simulink model "nms_3Dmodel_mld"  (R2019a)
settings: Solver=ode15s  StartTime=0.0  StopTime=7  FixedStep=1e-3  RelTol=1e-3  AbsTol=1e-4  EnableMultiTasking=on
InitFcn:
  | runScripts;
undefined symbols (not defined in the file or in its folder): ankle_height, c, c_jointstop, CtrlPar_FP, CtrlPar_FP_R, CtrlPar_LL, CtrlPar_St, CtrlPar_St_R, CtrlPar_Sw, CtrlPar_Sw_R, CtrlPar_theta0, CtrlPar_Tr, CtrlPar_Tr_R, D12_F, D12_S, D12_T, D12z_T, D13_F, D1G_F, D1G_HAT, D1G_S, D1G_T, D1Gy_F, d_fBall, d_fHeel, DeltaThRef, dt, eref, FmaxBFSH, FmaxGAS, FmaxGLU, FmaxHAB, FmaxHAD, FmaxHAM, FmaxHFL, FmaxRF, FmaxSOL, FmaxTA, FmaxVAS, In_F, In_HAT, In_S, In_T, init_a_tgt, init_a_tgtR, Inx_F, Inx_HAT, Inx_S, Inx_T, Iny_F, Iny_HAT, Iny_S, Iny_T, K, k_gn, k_gt, k_pressure, leg_l, LongDelay, LongLoopDelay ... (+139)
libraries: mblibv1 x89, simulink x44, simulink_extras x38
(part 7 of 13)

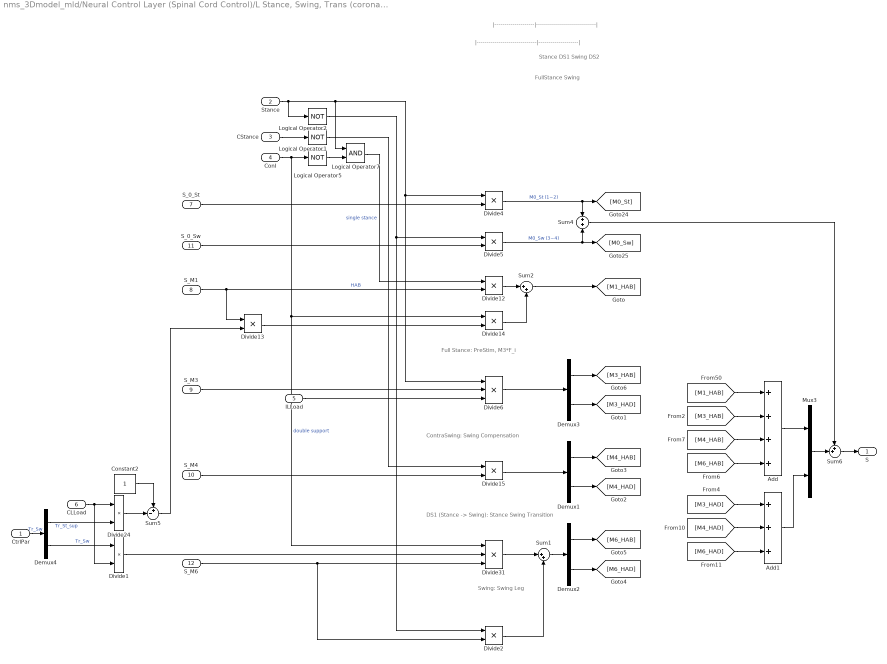
== system nms_3Dmodel_mld/Neural Control Layer (Spinal Cord Control)/L Stance, Swing, Trans (coronal) ==
  note: DS1 (Stance -> Swing):
      | Stance Swing Transition
  note: Swing:
      | Swing Leg
  note: Full Stance:
      | PreStim, M3*F_i
  note: Stance DS1 Swing DS2
  note: FullStance Swing
  note: |------------------------------|--------------------|
  note: |--------------------|------------------------------|
  note: ContraSwing:
      | Swing Compensation
  CtrlPar : Inport
  Stance : Inport  Port=2
  CStance : Inport  Port=3
  ConI : Inport  Port=4
  ILLoad : Inport  Port=5
  CLLoad : Inport  Port=6
  S_0_St : Inport  Port=7
  S_M1 : Inport  Port=8
  S_M3 : Inport  Port=9
  S_M4 : Inport  Port=10
  S_0_Sw : Inport  Port=11
  S_M6 : Inport  Port=12
  Add : Sum  Inputs=4
  Add1 : Sum  Inputs=3
  Constant2 : Constant
  Demux{1..4} (4 alike) : Demux  Outputs=2
  Divide{1..2,4..5,12..15,24} (9 alike) : Product
  Divide31 : Product  Inputs=3
  Divide6 : Product  Inputs=3
  Logical Operator1 : Logic  Operator=NOT  AllPortsSameDT=off  OutDataTypeStr=boolean
  Logical Operator2 : Logic  Operator=NOT  AllPortsSameDT=off  OutDataTypeStr=boolean
  Logical Operator5 : Logic  Operator=NOT  AllPortsSameDT=off  OutDataTypeStr=boolean
  Logical Operator7 : Logic  AllPortsSameDT=off  OutDataTypeStr=boolean
  Mux3 : Mux  Inputs=2
  Sum1 : Sum  Inputs=|++  SaturateOnIntegerOverflow=on  InputSameDT=on  OutDataTypeStr=Inherit: Same as first input
  Sum2 : Sum  Inputs=|++  SaturateOnIntegerOverflow=on  InputSameDT=on  OutDataTypeStr=Inherit: Same as first input
  Sum4 : Sum  SaturateOnIntegerOverflow=on  InputSameDT=on  OutDataTypeStr=Inherit: Same as first input
  Sum5 : Sum  Inputs=+-|  SaturateOnIntegerOverflow=on  InputSameDT=on  OutDataTypeStr=Inherit: Same as first input
  Sum6 : Sum  Inputs=++|  SaturateOnIntegerOverflow=on  InputSameDT=on  OutDataTypeStr=Inherit: Same as first input
  S : Outport  OutputWhenDisabled=reset  InitialOutput=0
  wires:
  CStance/1 -> Logical Operator1/1
  S_M4/1 -> Divide15/2
  Logical Operator1/1 -> Divide15/1
  CLLoad/1 -> Divide1/2, Divide24/1
  Divide1/1 -> Divide31/2
  ConI/1 -> Logical Operator5/1, Divide31/1, Divide14/1  "double support"
  Stance/1 -> Logical Operator2/1, Divide6/1, Divide4/1, Logical Operator7/1
  Logical Operator2/1 -> Divide2/1, Divide5/1
  Add/1 -> Mux3/1
  Add1/1 -> Mux3/2
  S_M3/1 -> Divide6/2
  ILLoad/1 -> Divide6/3
  S_0_St/1 -> Divide4/2
  S_0_Sw/1 -> Divide5/2
  Mux3/1 -> Sum6/2
  Sum6/1 -> S/1
  S_M6/1 -> Divide31/3, Divide2/2
  Divide4/1 -> Sum4/1, [M0_St]  "M0_St (1~2)"
  Divide5/1 -> Sum4/2, [M0_Sw]  "M0_Sw (3~4)"
  Divide31/1 -> Sum1/1
  Divide2/1 -> Sum1/2
  S_M1/1 -> Divide12/2, Divide13/1  "HAB"
  Divide12/1 -> Sum2/1
  Divide13/1 -> Divide14/2
  Divide14/1 -> Sum2/2
  Logical Operator5/1 -> Logical Operator7/2
  Logical Operator7/1 -> Divide12/1  "single stance"
  Divide24/1 -> Sum5/2
  Constant2/1 -> Sum5/1
  Sum5/1 -> Divide13/2
  CtrlPar/1 -> Demux4/1  "Tr_Sw"
  Demux4/1 -> Divide24/2  "Tr_St_sup"
  Demux4/2 -> Divide1/1  "Tr_Sw"
  Sum2/1 -> [M1_HAB]
  Divide6/1 -> Demux3/1
  Demux3/1 -> [M3_HAB]
  Demux3/2 -> [M3_HAD]
  Divide15/1 -> Demux1/1
  Demux1/1 -> [M4_HAB]
  Demux1/2 -> [M4_HAD]
  Demux2/1 -> [M6_HAB]
  Demux2/2 -> [M6_HAD]
  Sum1/1 -> Demux2/1
  Sum4/1 -> Sum6/1
  [M1_HAB] -> Add/1
  [M3_HAB] -> Add/2
  [M3_HAD] -> Add1/1
  [M4_HAB] -> Add/3
  [M6_HAB] -> Add/4
  [M4_HAD] -> Add1/2
  [M6_HAD] -> Add1/3

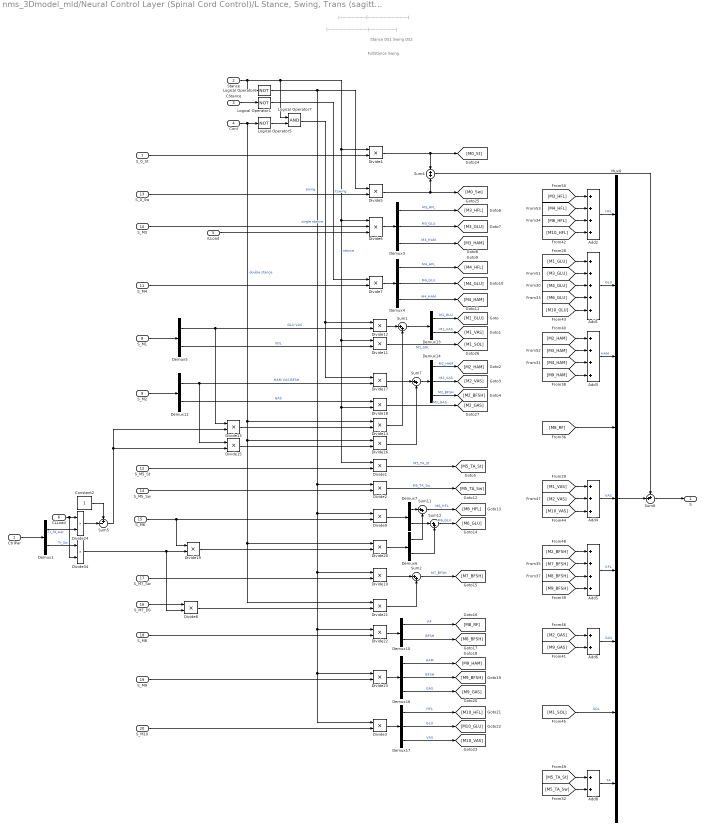
== system nms_3Dmodel_mld/Neural Control Layer (Spinal Cord Control)/L Stance, Swing, Trans (sagittal) ==
  note: Stance DS1 Swing DS2
  note: FullStance Swing
  note: |------------------------------|--------------------|
  note: |--------------------|------------------------------|
  CtrlPar : Inport
  Stance : Inport  Port=2
  CStance : Inport  Port=3
  ConI : Inport  Port=4
  ILLoad : Inport  Port=5
  CLLoad : Inport  Port=6
  S_0_St : Inport  Port=7
  S_M1 : Inport  Port=8
  S_M2 : Inport  Port=9
  S_M3 : Inport  Port=10
  S_M4 : Inport  Port=11
  S_M5_St : Inport  Port=12
  S_0_Sw : Inport  Port=13
  S_M5_Sw : Inport  Port=14
  S_M6 : Inport  Port=15
  S_M7_DS : Inport  Port=16
  S_M7_Sw : Inport  Port=17
  S_M8 : Inport  Port=18
  S_M9 : Inport  Port=19
  S_M10 : Inport  Port=20
  Add1 : Sum  Inputs=5
  Add2 : Sum  Inputs=4
  Add3 : Sum  Inputs=4
  Add4 : Sum  Inputs=3
  Add5 : Sum  Inputs=4
  Add6 : Sum  Inputs=2
  Add8 : Sum  Inputs=2
  Constant2 : Constant
  Demux{1,6..7,10,13} (5 alike) : Demux  Outputs=2
  Demux12 : Demux  Outputs=[3 1]
  Demux{3..4,14,16..17} (5 alike) : Demux  Outputs=3
  Demux5 : Demux  Outputs=[2 1]
  Divide{1..5,7..24,34} (24 alike) : Product
  Divide6 : Product  Inputs=3
  Logical Operator1 : Logic  Operator=NOT  AllPortsSameDT=off  OutDataTypeStr=boolean
  Logical Operator5 : Logic  Operator=NOT  AllPortsSameDT=off  OutDataTypeStr=boolean
  Logical Operator6 : Logic  Operator=NOT  AllPortsSameDT=off  OutDataTypeStr=boolean
  Logical Operator7 : Logic  AllPortsSameDT=off  OutDataTypeStr=boolean
  Mux6 : Mux  Inputs=9
  Sum{1..2,7,11..12} (5 alike) : Sum  Inputs=|++  SaturateOnIntegerOverflow=on  InputSameDT=on  OutDataTypeStr=Inherit: Same as first input
  Sum4 : Sum  SaturateOnIntegerOverflow=on  InputSameDT=on  OutDataTypeStr=Inherit: Same as first input
  Sum5 : Sum  Inputs=+-|  SaturateOnIntegerOverflow=on  InputSameDT=on  OutDataTypeStr=Inherit: Same as first input
  Sum6 : Sum  Inputs=++|  SaturateOnIntegerOverflow=on  InputSameDT=on  OutDataTypeStr=Inherit: Same as first input
  S : Outport  OutputWhenDisabled=reset  InitialOutput=0
  wires:
  CtrlPar/1 -> Demux1/1
  Stance/1 -> Logical Operator6/1, Logical Operator7/1, Divide4/1, Divide11/1, Divide18/2, Divide1/1, Divide6/1  "stance"
  ConI/1 -> Logical Operator5/1, Divide14/1, Divide16/1, Divide20/1, Divide21/1  "double stance"
  Logical Operator5/1 -> Logical Operator7/2
  S_M4/1 -> Divide7/2
  CStance/1 -> Logical Operator1/1
  Logical Operator1/1 -> Divide7/1  "Cswing"
  Demux1/1 -> Divide24/2  "Tr_St_sup"
  Divide24/1 -> Sum5/2
  Constant2/1 -> Sum5/1
  CLLoad/1 -> Divide24/1, Divide34/2
  Demux4/1 -> [M4_HFL]  "M4_HFL"
  Add2/1 -> Mux6/1  "HFL"
  Add1/1 -> Mux6/2  "GLU"
  Demux4/2 -> [M4_GLU]  "M4_GLU"
  Add3/1 -> Mux6/3  "HAM"
  Demux4/3 -> [M4_HAM]  "M4_HAM"
  Add4/1 -> Mux6/5  "VAS"
  Add5/1 -> Mux6/6  "KFL"
  Add6/1 -> Mux6/7  "GAS"
  Add8/1 -> Mux6/9  "TA"
  Demux1/2 -> Divide34/1  "Tr_Sw"
  Divide7/1 -> Demux4/1
  Logical Operator7/1 -> Divide12/1, Divide17/1  "single stance"
  Divide34/1 -> Divide19/2, Divide8/2
  Logical Operator6/1 -> Divide5/1, Divide2/1, Divide9/1, Divide10/1, Divide3/1, Divide23/1, Divide22/1  "swing"
  Mux6/1 -> Sum6/2
  Sum6/1 -> S/1
  Sum4/1 -> Sum6/1
  S_0_Sw/1 -> Divide5/2
  S_0_St/1 -> Divide4/2
  Divide5/1 -> [M0_Sw], Sum4/2
  Divide4/1 -> Sum4/1, [M0_St]
  S_M1/1 -> Demux5/1
  S_M2/1 -> Demux12/1
  Demux5/1 -> Divide12/2, Divide13/1  "GLU VAS"
  Demux5/2 -> Divide11/2  "SOL"
  Divide12/1 -> Sum1/1
  Divide13/1 -> Divide14/2
  Divide14/1 -> Sum1/2
  Divide16/1 -> Sum7/2
  Divide15/1 -> Divide16/2
  Sum1/1 -> Demux13/1
  Demux13/1 -> [M1_GLU]  "M1_GLU"
  Demux13/2 -> [M1_VAS]  "M1_VAS"
  Demux12/1 -> Divide17/2, Divide15/1  "HAM VAS BFSH"
  Divide17/1 -> Sum7/1
  Sum7/1 -> Demux14/1
  Demux14/1 -> [M2_HAM]  "M2_HAM"
  Demux14/2 -> [M2_VAS]  "M2_VAS"
  Demux14/3 -> [M2_BFSH]  "M2_BFSH"
  Demux12/2 -> Divide18/1  "GAS"
  Divide18/1 -> [M2_GAS]  "M2_GAS"
  S_M5_St/1 -> Divide1/2
  Divide1/1 -> [M5_TA_St]  "M5_TA_St"
  Divide11/1 -> [M1_SOL]  "M1_SOL"
  S_M3/1 -> Divide6/2
  ILLoad/1 -> Divide6/3
  Divide6/1 -> Demux3/1
  Demux3/1 -> [M3_HFL]  "M3_HFL"
  Demux3/2 -> [M3_GLU]  "M3_GLU"
  Demux3/3 -> [M3_HAM]  "M3_HAM"
  S_M5_Sw/1 -> Divide2/2
  Divide2/1 -> [M5_TA_Sw]  "M5_TA_Sw"
  S_M6/1 -> Divide9/2, Divide19/1
  Divide9/1 -> Demux7/1
  Demux7/2 -> Sum12/1
  Divide20/1 -> Demux6/1
  Demux6/1 -> Sum11/2
  Demux6/2 -> Sum12/2
  Demux7/1 -> Sum11/1
  Divide19/1 -> Divide20/2
  Sum11/1 -> [M6_HFL]  "M6_HFL"
  Sum12/1 -> [M6_GLU]  "M6_GLU"
  Divide10/1 -> Sum2/1
  Divide21/1 -> Sum2/2
  Sum5/1 -> Divide13/2, Divide15/2
  S_M7_Sw/1 -> Divide10/2
  Divide8/1 -> Divide21/2
  S_M7_DS/1 -> Divide8/1
  Sum2/1 -> [M7_BFSH]  "M7_BFSH"
  S_M8/1 -> Divide22/2
  Divide22/1 -> Demux10/1
  S_M9/1 -> Divide23/2
  Divide23/1 -> Demux16/1
  S_M10/1 -> Divide3/2
  Divide3/1 -> Demux17/1
  Demux10/2 -> [M8_BFSH]  "BFSH"
  Demux10/1 -> [M8_RF]  "RF"
  Demux16/1 -> [M9_HAM]  "HAM"
  Demux16/2 -> [M9_BFSH]  "BFSH"
  Demux16/3 -> [M9_GAS]  "GAS"
  Demux17/1 -> [M10_HFL]  "HFL"
  Demux17/2 -> [M10_GLU]  "GLU"
  Demux17/3 -> [M10_VAS]  "VAS"
  [M1_GLU] -> Add1/1
  [M3_GLU] -> Add1/2
  [M4_GLU] -> Add1/3
  [M6_GLU] -> Add1/4
  [M10_GLU] -> Add1/5
  [M1_VAS] -> Add4/1
  [M2_HAM] -> Add3/1
  [M2_VAS] -> Add4/2
  [M2_BFSH] -> Add5/1
  [M2_GAS] -> Add6/1
  [M3_HFL] -> Add2/1
  [M3_HAM] -> Add3/2
  [M4_HFL] -> Add2/2
  [M4_HAM] -> Add3/3
  [M5_TA_St] -> Add8/1
  [M5_TA_Sw] -> Add8/2
  [M6_HFL] -> Add2/3
  [M7_BFSH] -> Add5/2
  [M9_BFSH] -> Add5/4
  [M8_BFSH] -> Add5/3
  [M8_RF] -> Mux6/4
  [M9_HAM] -> Add3/4
  [M9_GAS] -> Add6/2
  [M10_HFL] -> Add2/4
  [M10_VAS] -> Add4/3
  [M1_SOL] -> Mux6/8  "SOL"

== system nms_3Dmodel_mld/Neural Control Layer (Spinal Cord Control)/L Swing Phase (coronal) ==
  note: Left Swing Phase Control
  note: M6: swing hip
  CtrlPar : Inport
  R_a_tgt : Inport  Port=2
  LceHAD : Inport  Port=3
  LceHAB : Inport  Port=4
  Enable : EnablePort  StatesWhenEnabling=reset  ZeroCross=off
  Constant1 : Constant
  Constant5 : Constant
  Demux4 : Demux  Outputs=6
  Divide{1..2,5,22} (4 alike) : Product
  Mux1 : Mux  Inputs=2
  R_parSwPreS : Selector  InputPortWidth=R_Sw_i  IndexOptions=Index vector (dialog)  Indices=R_parSw_PreS_i  OutputSizes=1
  R_parSw_M6 : Selector  InputPortWidth=R_Sw_i  IndexOptions=Index vector (dialog)  Indices=R_parSw_M6_i  OutputSizes=1
  Sum1 : Sum  Inputs=-+|  SaturateOnIntegerOverflow=on  InputSameDT=on  OutDataTypeStr=Inherit: Same as first input
  Sum10 : Sum  Inputs=++|  SaturateOnIntegerOverflow=on  InputSameDT=on  OutDataTypeStr=Inherit: Same as first input
  Sum13 : Sum  Inputs=|+-  SaturateOnIntegerOverflow=on  InputSameDT=on  OutDataTypeStr=Inherit: Same as first input
  Sum2 : Sum  Inputs=-+|  SaturateOnIntegerOverflow=on  InputSameDT=on  OutDataTypeStr=Inherit: Same as first input
  Sum3 : Sum  Inputs=+-|  SaturateOnIntegerOverflow=on  InputSameDT=on  OutDataTypeStr=Inherit: Same as first input
  Sum4 : Sum  Inputs=|+-  SaturateOnIntegerOverflow=on  InputSameDT=on  OutDataTypeStr=Inherit: Same as first input
  positive half1 : Saturate  UpperLimit=inf  LowerLimit=0  ZeroCross=off
  positive half2 : Saturate  UpperLimit=inf  LowerLimit=0  ZeroCross=off
  S_0_Sw : Outport  OutputWhenDisabled=reset  InitialOutput=0
  S_M6 [HAB HAD] : Outport  Port=2  OutputWhenDisabled=reset  InitialOutput=0
  wires:
  R_parSwPreS/1 -> S_0_Sw/1
  CtrlPar/1 -> R_parSwPreS/1, R_parSw_M6/1
  R_parSw_M6/1 -> Demux4/1
  Constant5/1 -> Sum10/1
  Demux4/2 -> Sum13/2  "aRef_HAB"
  Sum13/1 -> Divide22/2
  Demux4/1 -> Divide22/1  "a2lopt_HAB"
  Divide22/1 -> Sum10/2
  Sum10/1 -> Sum1/1  "lceOffHAB"
  Sum1/1 -> positive half2/1
  positive half2/1 -> Divide5/1
  Demux4/3 -> Divide5/2  "LGain_HAB"
  Constant1/1 -> Sum3/1
  R_a_tgt/1 -> Sum4/1, Sum13/1
  Demux4/5 -> Sum4/2  "aRef_HAD"
  Sum4/1 -> Divide1/2
  Demux4/4 -> Divide1/1  "a2lopt_HAD"
  Divide1/1 -> Sum3/2
  Sum3/1 -> Sum2/1  "lceOffHAD"
  Sum2/1 -> positive half1/1
  positive half1/1 -> Divide2/1
  Demux4/6 -> Divide2/2  "LGain_HAD"
  LceHAB/1 -> Sum1/2
  LceHAD/1 -> Sum2/2
  Divide5/1 -> Mux1/1  "HAB"
  Divide2/1 -> Mux1/2  "HAD"
  Mux1/1 -> S_M6 [HAB HAD]/1

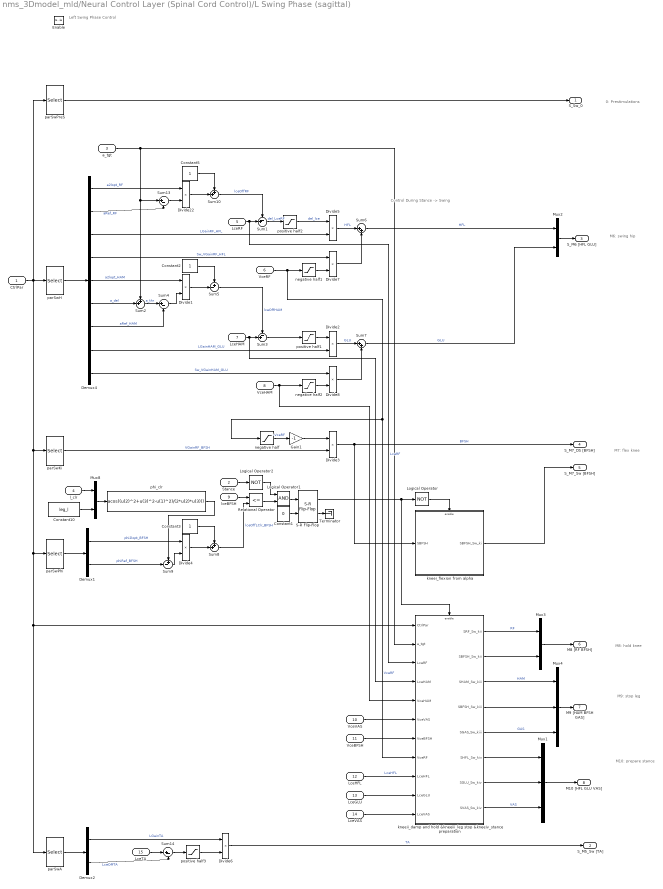
== system nms_3Dmodel_mld/Neural Control Layer (Spinal Cord Control)/L Swing Phase (sagittal) ==
  note: Left Swing Phase Control
  note: Control During Stance -> Swing
  note: 0: Prestimulations
  note: M6: swing hip
  note: M7: flex knee
  note: M8: hold knee
  note: M9: stop leg
  note: M10: prepare stance
  CtrlPar : Inport
  Stance : Inport  Port=2
  a_tgt : Inport  Port=3
  l_clr : Inport  Port=4
  LceRF : Inport  Port=5
  VceRF : Inport  Port=6
  LceHAM : Inport  Port=7
  VceHAM : Inport  Port=8
  lceBFSH : Inport  Port=9
  VceVAS : Inport  Port=10
  VceBFSH : Inport  Port=11
  LceHFL : Inport  Port=12
  LceGLU : Inport  Port=13
  LceVAS : Inport  Port=14
  LceTA : Inport  Port=15
  Enable : EnablePort  StatesWhenEnabling=reset  ZeroCross=off
  Constant1 : Constant  Value=0  OutDataTypeStr=boolean
  Constant10 : Constant  Value=leg_l
  Constant2 : Constant
  Constant3 : Constant
  Constant5 : Constant
  Demux1 : Demux  Outputs=2
  Demux2 : Demux  Outputs=2
  Demux4 : Demux  Outputs=9
  Divide{1..8,22} (9 alike) : Product
  Gain1 : Gain  Gain=-1
  Logical Operator : Logic  Operator=NOT  AllPortsSameDT=off  OutDataTypeStr=boolean
  Logical Operator1 : Logic  AllPortsSameDT=off  OutDataTypeStr=boolean
  Logical Operator2 : Logic  Operator=NOT  AllPortsSameDT=off  OutDataTypeStr=boolean
  Mux1 : Mux  Inputs=3
  Mux2 : Mux  Inputs=2
  Mux3 : Mux  Inputs=2
  Mux4 : Mux  Inputs=3
  Mux8 : Mux  Inputs=2
  Relational Operator : RelationalOperator  Operator=<=  OutDataTypeStr=boolean  ZeroCross=off  RndMeth=Nearest
  S-R Flip-Flop : simulink_extras/Flip Flops/S-R Flip-Flop  initial_condition=0
  Sum1 : Sum  Inputs=-+|  SaturateOnIntegerOverflow=on  InputSameDT=on  OutDataTypeStr=Inherit: Same as first input
  Sum10 : Sum  Inputs=++|  SaturateOnIntegerOverflow=on  InputSameDT=on  OutDataTypeStr=Inherit: Same as first input
  Sum13 : Sum  Inputs=|+-  SaturateOnIntegerOverflow=on  InputSameDT=on  OutDataTypeStr=Inherit: Same as first input
  Sum14 : Sum  Inputs=|+-  SaturateOnIntegerOverflow=on  InputSameDT=on  OutDataTypeStr=Inherit: Same as first input
  Sum2 : Sum  Inputs=++|  SaturateOnIntegerOverflow=on  InputSameDT=on  OutDataTypeStr=Inherit: Same as first input
  Sum3 : Sum  Inputs=-+|  SaturateOnIntegerOverflow=on  InputSameDT=on  OutDataTypeStr=Inherit: Same as first input
  Sum4 : Sum  Inputs=|+-  SaturateOnIntegerOverflow=on  InputSameDT=on  OutDataTypeStr=Inherit: Same as first input
  Sum5 : Sum  Inputs=+-|  SaturateOnIntegerOverflow=on  InputSameDT=on  OutDataTypeStr=Inherit: Same as first input
  Sum6 : Sum  Inputs=|++  SaturateOnIntegerOverflow=on  InputSameDT=on  OutDataTypeStr=Inherit: Same as first input
  Sum7 : Sum  Inputs=|++  SaturateOnIntegerOverflow=on  InputSameDT=on  OutDataTypeStr=Inherit: Same as first input
  Sum8 : Sum  Inputs=++|  SaturateOnIntegerOverflow=on  InputSameDT=on  OutDataTypeStr=Inherit: Same as first input
  Sum9 : Sum  Inputs=+-|  SaturateOnIntegerOverflow=on  InputSameDT=on  OutDataTypeStr=Inherit: Same as first input
  Terminator : Terminator
  kneei_flexion from alpha : Subsystem  TreatAsAtomicUnit=on
  kneeii_damp and hold &kneeiii_leg stop &kneeiv_stance preparation : Subsystem  TreatAsAtomicUnit=on
  negative half : Saturate  UpperLimit=0  LowerLimit=-inf  ZeroCross=off
  negative half1 : Saturate  UpperLimit=0  LowerLimit=-inf  ZeroCross=off
  negative half2 : Saturate  UpperLimit=0  LowerLimit=-inf  ZeroCross=off
  parSwA : Selector  InputPortWidth=Sw_i  IndexOptions=Index vector (dialog)  Indices=parSwA_i  OutputSizes=1
  parSwH : Selector  InputPortWidth=Sw_i  IndexOptions=Index vector (dialog)  Indices=parSwH_i  OutputSizes=1
  parSwKi : Selector  InputPortWidth=Sw_i  IndexOptions=Index vector (dialog)  Indices=parSwKi_i  OutputSizes=1
  parSwPhi : Selector  InputPortWidth=Sw_i  IndexOptions=Index vector (dialog)  Indices=parSwPhi_i  OutputSizes=1
  parSwPreS : Selector  InputPortWidth=Sw_i  IndexOptions=Index vector (dialog)  Indices=parSwPreS_i  OutputSizes=1
  phi_clr : Fcn  Expr=acos((u(2)^2+u(3)^2-u(1)^2)/(2*u(2)*u(3)))
  positive half1 : Saturate  UpperLimit=inf  LowerLimit=0  ZeroCross=off
  positive half2 : Saturate  UpperLimit=inf  LowerLimit=0  ZeroCross=off
  positive half3 : Saturate  UpperLimit=inf  LowerLimit=0  ZeroCross=off
  S_Sw_0 : Outport  OutputWhenDisabled=reset  InitialOutput=0
  S_M5_Sw [TA] : Outport  Port=2  OutputWhenDisabled=reset  InitialOutput=0
  S_M6 [HFL GLU] : Outport  Port=3  OutputWhenDisabled=reset  InitialOutput=0
  S_M7_DS [BFSH] : Outport  Port=4  OutputWhenDisabled=reset  InitialOutput=0
  S_M7_Sw [BFSH] : Outport  Port=5  OutputWhenDisabled=reset  InitialOutput=0
  M8 [RF BFSH] : Outport  Port=6  OutputWhenDisabled=reset  InitialOutput=0
  M9 [HAM BFSH GAS] : Outport  Port=7  OutputWhenDisabled=reset  InitialOutput=0
  M10 [HFL GLU VAS] : Outport  Port=8  OutputWhenDisabled=reset  InitialOutput=0
  wires:
  CtrlPar/1 -> parSwH/1, parSwKi/1, parSwPhi/1, kneeii_damp and hold &kneeiii_leg stop &kneeiv_stance preparation/1(CtrlPar), parSwA/1, parSwPreS/1
  parSwH/1 -> Demux4/1
  Constant5/1 -> Sum10/1
  a_tgt/1 -> Sum13/1, Sum2/1, kneeii_damp and hold &kneeiii_leg stop &kneeiv_stance preparation/2(a_tgt)
  Demux4/2 -> Sum13/2  "aRef_RF"
  Sum13/1 -> Divide22/2
  Demux4/1 -> Divide22/1  "a2lopt_RF"
  Divide22/1 -> Sum10/2
  Sum10/1 -> Sum1/1  "lceOffRF"
  Sum1/1 -> positive half2/1  "del_LceRF"
  positive half2/1 -> Divide5/1  "del_lce"
  Demux4/3 -> Divide5/2  "LGainRF_HFL"
  Demux4/6 -> Sum2/2  "a_del"
  Sum2/1 -> Sum4/1  "a_thr"
  Demux4/7 -> Sum4/2  "aRef_HAM"
  Sum4/1 -> Divide1/2
  Demux4/5 -> Divide1/1  "a2lopt_HAM"
  Constant2/1 -> Sum5/1
  Divide1/1 -> Sum5/2
  Sum3/1 -> positive half1/1
  positive half1/1 -> Divide2/1
  Demux4/8 -> Divide2/2  "LGainHAM_GLU"
  Sum5/1 -> Sum3/1  "lceOffHAM"
  LceHAM/1 -> Sum3/2, kneeii_damp and hold &kneeiii_leg stop &kneeiv_stance preparation/4(LceHAM)
  Gain1/1 -> Divide3/1
  negative half/1 -> Gain1/1  "-VceRF"
  parSwKi/1 -> Divide3/2  "VGainRF_BFSH"
  Divide3/1 -> kneei_flexion from alpha/1(SBFSH), S_M7_DS [BFSH]/1  "BFSH"
  Constant1/1 -> S-R Flip-Flop/2
  S-R Flip-Flop/2 -> Terminator/1
  S-R Flip-Flop/1 -> Logical Operator/1, kneeii_damp and hold &kneeiii_leg stop &kneeiv_stance preparation/Enable
  Logical Operator/1 -> kneei_flexion from alpha/Enable
  lceBFSH/1 -> Relational Operator/1
  Mux8/1 -> phi_clr/1
  l_clr/1 -> Mux8/1
  Constant10/1 -> Mux8/2
  parSwPhi/1 -> Demux1/1
  Sum9/1 -> Divide4/2
  Demux1/1 -> Divide4/1  "phi2lopt_BFSH"
  Demux1/2 -> Sum9/2  "phiRef_BFSH"
  phi_clr/1 -> Sum9/1
  Constant3/1 -> Sum8/1
  Divide4/1 -> Sum8/2
  Sum8/1 -> Relational Operator/2  "lceOffLClr_BFSH"
  VceBFSH/1 -> kneeii_damp and hold &kneeiii_leg stop &kneeiv_stance preparation/7(VceBFSH)
  LceHFL/1 -> kneeii_damp and hold &kneeiii_leg stop &kneeiv_stance preparation/9(LceHFL)  "LceHFL"
  LceGLU/1 -> kneeii_damp and hold &kneeiii_leg stop &kneeiv_stance preparation/10(LceGLU)
  LceVAS/1 -> kneeii_damp and hold &kneeiii_leg stop &kneeiv_stance preparation/11(LceVAS)
  kneeii_damp and hold &kneeiii_leg stop &kneeiv_stance preparation/6(SHFL_Sw_kiv) -> Mux1/1
  kneeii_damp and hold &kneeiii_leg stop &kneeiv_stance preparation/7(SGLU_Sw_kiv) -> Mux1/2
  kneei_flexion from alpha/1(SBFSH_Sw_ki) -> S_M7_Sw [BFSH]/1
  kneeii_damp and hold &kneeiii_leg stop &kneeiv_stance preparation/2(SBFSH_Sw_kii) -> Mux3/2
  kneeii_damp and hold &kneeiii_leg stop &kneeiv_stance preparation/4(SBFSH_Sw_kiii) -> Mux4/2
  parSwA/1 -> Demux2/1
  Demux2/1 -> Divide6/1  "LGainTA"
  Sum14/1 -> positive half3/1
  LceTA/1 -> Sum14/1
  positive half3/1 -> Divide6/2
  Demux2/2 -> Sum14/2  "LceOffTA"
  Logical Operator1/1 -> S-R Flip-Flop/1
  Relational Operator/1 -> Logical Operator1/2
  Stance/1 -> Logical Operator2/1
  Logical Operator2/1 -> Logical Operator1/1
  parSwPreS/1 -> S_Sw_0/1
  kneeii_damp and hold &kneeiii_leg stop &kneeiv_stance preparation/3(SHAM_Sw_kiii) -> Mux4/1  "HAM"
  kneeii_damp and hold &kneeiii_leg stop &kneeiv_stance preparation/1(SRF_Sw_kii) -> Mux3/1  "RF"
  kneeii_damp and hold &kneeiii_leg stop &kneeiv_stance preparation/8(SVAS_Sw_kiv) -> Mux1/3  "VAS"
  Divide6/1 -> S_M5_Sw [TA]/1  "TA"
  kneeii_damp and hold &kneeiii_leg stop &kneeiv_stance preparation/5(SGAS_Sw_kiii) -> Mux4/3  "GAS"
  Mux2/1 -> S_M6 [HFL GLU]/1
  Mux3/1 -> M8 [RF BFSH]/1
  Mux4/1 -> M9 [HAM BFSH GAS]/1
  Mux1/1 -> M10 [HFL GLU VAS]/1
  LceRF/1 -> Sum1/2, kneeii_damp and hold &kneeiii_leg stop &kneeiv_stance preparation/3(LceRF)  "LceRF"
  VceVAS/1 -> kneeii_damp and hold &kneeiii_leg stop &kneeiv_stance preparation/6(VceVAS)
  Demux4/4 -> Divide7/1  "Sw_VGainRF_HFL"
  Demux4/9 -> Divide8/1  "Sw_VGainHAM_GLU"
  VceRF/1 -> kneeii_damp and hold &kneeiii_leg stop &kneeiv_stance preparation/8(VceRF), negative half/1, negative half1/1  "VceRF"
  VceHAM/1 -> kneeii_damp and hold &kneeiii_leg stop &kneeiv_stance preparation/5(VceHAM), negative half2/1
  Divide5/1 -> Sum6/1  "HFL"
  Divide7/1 -> Sum6/2
  Sum6/1 -> Mux2/1  "HFL"
  negative half1/1 -> Divide7/2
  negative half2/1 -> Divide8/2
  Divide2/1 -> Sum7/1  "GLU"
  Sum7/1 -> Mux2/2  "GLU"
  Divide8/1 -> Sum7/2

== system nms_3Dmodel_mld/Neural Control Layer (Spinal Cord Control)/R Stance Phase (coronal) ==
  note: Left Stance Phase Control
  note: M3: balance trunk
  note: M4: compensate swing leg
  CtrlPar : Inport
  theta_tgt [rad] : Inport  Port=2
  theta dtheta [rad rad/s] : Inport  Port=3
  CSwingStim : Inport  Port=4
  FmHAB : Inport  Port=5
  Enable : EnablePort  StatesWhenEnabling=reset  ZeroCross=off
  Demux1 : Demux  Outputs=2
  Demux2 : Demux
  Demux7 : Demux  Outputs=2
  Demux8 : Demux  Outputs=2
  Divide{1,4,6..7,9,14..15} (7 alike) : Product
  Gain2 : Gain  Gain=-1
  Gain3 : Gain  Gain=-1
  Mux1 : Mux  Inputs=2
  Mux2 : Mux  Inputs=2
  R_parSt_M1 : Selector  InputPortWidth=R_St_i  IndexOptions=Index vector (dialog)  Indices=R_parSt_M1_i  OutputSizes=1
  R_parSt_M3 : Selector  InputPortWidth=R_St_i  IndexOptions=Index vector (dialog)  Indices=R_parSt_M3_i  OutputSizes=1
  R_parSt_M4 : Selector  InputPortWidth=R_St_i  IndexOptions=Index vector (dialog)  Indices=R_parSt_M4_i  OutputSizes=1
  R_parSt_PreS : Selector  InputPortWidth=R_St_i  IndexOptions=Index vector (dialog)  Indices=R_parSt_PreS_i  OutputSizes=1
  Sum4 : Sum  Inputs=-+|  SaturateOnIntegerOverflow=on  InputSameDT=on  OutDataTypeStr=Inherit: Same as first input
  Sum5 : Sum  Inputs=|++  SaturateOnIntegerOverflow=on  InputSameDT=on  OutDataTypeStr=Inherit: Same as first input
  Sum6 : Sum  Inputs=|++  SaturateOnIntegerOverflow=on  InputSameDT=on  OutDataTypeStr=Inherit: Same as first input
  positive half1 : Saturate  UpperLimit=inf  LowerLimit=0  ZeroCross=off
  positive half2 : Saturate  UpperLimit=inf  LowerLimit=0  ZeroCross=off
  S_0_St : Outport  OutputWhenDisabled=reset  InitialOutput=0
  S_M1 [HAB] : Outport  Port=2  OutputWhenDisabled=reset  InitialOutput=0
  S_M3 [HAB HAD] : Outport  Port=3  OutputWhenDisabled=reset  InitialOutput=0
  S_M4 [HAB HAD] : Outport  Port=4  OutputWhenDisabled=reset  InitialOutput=0
  wires:
  theta dtheta [rad rad/s]/1 -> Demux7/1
  Demux7/1 -> Sum4/2  "theta"
  Demux7/2 -> Gain3/1, Divide15/1  "dtheta"
  theta_tgt [rad]/1 -> Sum4/1
  Sum4/1 -> Gain2/1, Divide14/1
  Demux2/1 -> Divide4/2  "GainTh_HAB"
  Demux2/2 -> Divide6/2  "GainDTh_HAB"
  Demux2/3 -> Divide14/2  "GainTh_HAD"
  Demux2/4 -> Divide15/2  "GainDTh_HAD"
  Gain2/1 -> Divide4/1
  Gain3/1 -> Divide6/1
  Divide4/1 -> Sum5/1
  Divide6/1 -> Sum5/2
  Divide14/1 -> Sum6/1
  Divide15/1 -> Sum6/2
  Sum5/1 -> positive half1/1  "HAB"
  Sum6/1 -> positive half2/1  "HAD"
  Mux1/1 -> S_M3 [HAB HAD]/1
  R_parSt_PreS/1 -> S_0_St/1
  CtrlPar/1 -> R_parSt_PreS/1, R_parSt_M4/1, R_parSt_M3/1, R_parSt_M1/1
  R_parSt_M3/1 -> Demux2/1
  CSwingStim/1 -> Demux8/1
  Mux2/1 -> S_M4 [HAB HAD]/1
  Demux8/1 -> Divide9/2  "Stim_CHAB"
  Demux8/2 -> Divide1/2  "Stim_CHAD"
  R_parSt_M4/1 -> Demux1/1
  Demux1/1 -> Divide9/1  "SGainCHAB_HAB"
  Divide9/1 -> Mux2/1  "HAB"
  Demux1/2 -> Divide1/1  "SGainCHAD_HAD"
  Divide1/1 -> Mux2/2  "HAD"
  positive half1/1 -> Mux1/1
  positive half2/1 -> Mux1/2
  R_parSt_M1/1 -> Divide7/1  "FGain_HAB"
  Divide7/1 -> S_M1 [HAB]/1  "HAB"
  FmHAB/1 -> Divide7/2

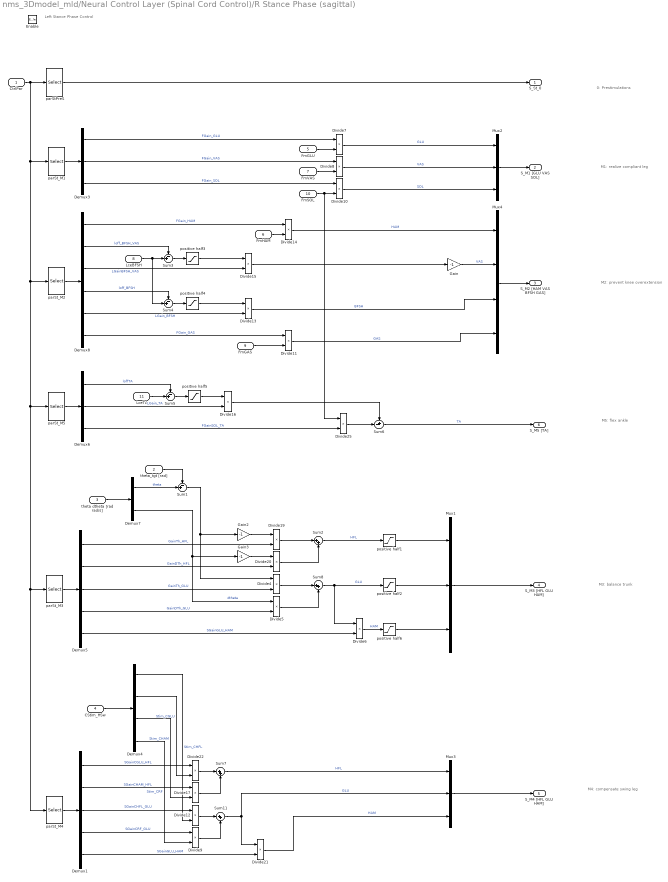
== system nms_3Dmodel_mld/Neural Control Layer (Spinal Cord Control)/R Stance Phase (sagittal) ==
  note: Left Stance Phase Control
  note: 0: Prestimulations
  note: M1: realize compliant leg
  note: M2: prevent knee overextension
  note: M5: flex ankle
  note: M3: balance trunk
  note: M4: compensate swing leg
  CtrlPar : Inport
  theta_tgt [rad] : Inport  Port=2
  theta dtheta [rad rad/s] : Inport  Port=3
  CStim_HSw : Inport  Port=4
  FmGLU : Inport  Port=5
  FmHAM : Inport  Port=6
  FmVAS : Inport  Port=7
  LceBFSH : Inport  Port=8
  FmGAS : Inport  Port=9
  FmSOL : Inport  Port=10
  LceTA : Inport  Port=11
  Enable : EnablePort  StatesWhenEnabling=reset  ZeroCross=off
  Demux1 : Demux  Outputs=5
  Demux3 : Demux  Outputs=3
  Demux4 : Demux
  Demux5 : Demux  Outputs=5
  Demux6 : Demux  Outputs=3
  Demux7 : Demux  Outputs=2
  Demux8 : Demux  Outputs=6
  Divide{4..17,19..22,25} (19 alike) : Product
  Gain : Gain  Gain=-1
  Gain2 : Gain  Gain=-1
  Gain3 : Gain  Gain=-1
  Mux1 : Mux  Inputs=3
  Mux2 : Mux  Inputs=3
  Mux3 : Mux  Inputs=3
  Mux4 : Mux
  Sum{1,3..5} (4 alike) : Sum  Inputs=-+|  SaturateOnIntegerOverflow=on  InputSameDT=on  OutDataTypeStr=Inherit: Same as first input
  Sum{2,7..8,11} (4 alike) : Sum  Inputs=|++  SaturateOnIntegerOverflow=on  InputSameDT=on  OutDataTypeStr=Inherit: Same as first input
  Sum6 : Sum  Inputs=+-|  SaturateOnIntegerOverflow=on  InputSameDT=on  OutDataTypeStr=Inherit: Same as first input
  parStPreS : Selector  InputPortWidth=St_i  IndexOptions=Index vector (dialog)  Indices=parSt_PreS_i  OutputSizes=1
  parSt_M1 : Selector  InputPortWidth=St_i  IndexOptions=Index vector (dialog)  Indices=parSt_M1_i  OutputSizes=1
  parSt_M2 : Selector  InputPortWidth=St_i  IndexOptions=Index vector (dialog)  Indices=parSt_M2_i  OutputSizes=1
  parSt_M3 : Selector  InputPortWidth=St_i  IndexOptions=Index vector (dialog)  Indices=parSt_M3_i  OutputSizes=1
  parSt_M4 : Selector  InputPortWidth=St_i  IndexOptions=Index vector (dialog)  Indices=parSt_M4_i  OutputSizes=1
  parSt_M5 : Selector  InputPortWidth=St_i  IndexOptions=Index vector (dialog)  Indices=parSt_M5_i  OutputSizes=1
  positive half{1..6} (6 alike) : Saturate  UpperLimit=inf  LowerLimit=0  ZeroCross=off
  S_St_0 : Outport  OutputWhenDisabled=reset  InitialOutput=0
  S_M1 [GLU VAS SOL] : Outport  Port=2  OutputWhenDisabled=reset  InitialOutput=0
  S_M2 [HAM VAS BFSH GAS] : Outport  Port=3  OutputWhenDisabled=reset  InitialOutput=0
  S_M3 [HFL GLU HAM] : Outport  Port=4  OutputWhenDisabled=reset  InitialOutput=0
  S_M4 [HFL GLU HAM] : Outport  Port=5  OutputWhenDisabled=reset  InitialOutput=0
  S_M5 [TA] : Outport  Port=6  OutputWhenDisabled=reset  InitialOutput=0
  wires:
  CtrlPar/1 -> parStPreS/1, parSt_M1/1, parSt_M2/1, parSt_M5/1, parSt_M3/1, parSt_M4/1
  parStPreS/1 -> S_St_0/1
  parSt_M1/1 -> Demux3/1
  Demux3/2 -> Divide8/1  "FGain_VAS"
  Demux3/3 -> Divide10/1  "FGain_SOL"
  Divide10/1 -> Mux2/3  "SOL"
  Divide8/1 -> Mux2/2  "VAS"
  Demux3/1 -> Divide7/1  "FGain_GLU"
  Divide7/1 -> Mux2/1  "GLU"
  Mux2/1 -> S_M1 [GLU VAS SOL]/1
  FmGLU/1 -> Divide7/2
  FmVAS/1 -> Divide8/2
  FmSOL/1 -> Divide10/2, Divide25/1
  parSt_M2/1 -> Demux8/1
  Sum3/1 -> positive half3/1
  Demux8/3 -> Divide15/2  "LGainBFSH_VAS"
  Demux8/5 -> Divide13/2  "LGain_BFSH"
  Demux8/6 -> Divide11/1  "FGain_GAS"
  positive half3/1 -> Divide15/1
  Demux8/2 -> Sum3/1  "loff_BFSH_VAS"
  Divide15/1 -> Gain/1
  Divide13/1 -> Mux4/3  "BFSH"
  Divide11/1 -> Mux4/4  "GAS"
  Demux8/1 -> Divide14/1  "FGain_HAM"
  Divide14/1 -> Mux4/1  "HAM"
  Gain/1 -> Mux4/2  "VAS"
  Sum4/1 -> positive half4/1
  positive half4/1 -> Divide13/1
  Demux8/4 -> Sum4/1  "loff_BFSH"
  FmHAM/1 -> Divide14/2
  LceBFSH/1 -> Sum3/2, Sum4/2
  FmGAS/1 -> Divide11/2
  Sum5/1 -> positive half5/1
  positive half5/1 -> Divide16/1
  Divide16/1 -> Sum6/1
  Divide25/1 -> Sum6/2
  parSt_M5/1 -> Demux6/1
  Demux6/1 -> Sum5/1  "loffTA"
  Demux6/2 -> Divide16/2  "LGain_TA"
  Demux6/3 -> Divide25/2  "FGainSOL_TA"
  Sum6/1 -> S_M5 [TA]/1  "TA"
  LceTA/1 -> Sum5/2
  Mux4/1 -> S_M2 [HAM VAS BFSH GAS]/1
  parSt_M3/1 -> Demux5/1
  Demux5/1 -> Divide19/2  "GainTh_HFL"
  Demux5/2 -> Divide20/2  "GainDTh_HFL"
  Demux5/3 -> Divide4/2  "GainTh_GLU"
  Demux5/4 -> Divide5/2  "GainDTh_GLU"
  theta dtheta [rad rad/s]/1 -> Demux7/1
  Demux7/1 -> Sum1/2  "theta"
  Demux7/2 -> Gain3/1, Divide5/1  "dtheta"
  Sum1/1 -> Gain2/1, Divide4/1
  Gain2/1 -> Divide19/1
  Gain3/1 -> Divide20/1
  Divide19/1 -> Sum2/1
  Divide20/1 -> Sum2/2
  Divide4/1 -> Sum8/1
  Divide5/1 -> Sum8/2
  Sum2/1 -> positive half1/1  "HFL"
  Sum8/1 -> Divide6/1, positive half2/1  "GLU"
  Mux1/1 -> S_M3 [HFL GLU HAM]/1
  Demux5/5 -> Divide6/2  "SGainGLU_HAM"
  Divide6/1 -> positive half6/1  "HAM"
  theta_tgt [rad]/1 -> Sum1/1
  positive half1/1 -> Mux1/1
  positive half2/1 -> Mux1/2
  positive half6/1 -> Mux1/3
  parSt_M4/1 -> Demux1/1
  Demux1/1 -> Divide22/1  "SGainCGLU_HFL"
  Demux1/3 -> Divide12/1  "SGainCHFL_GLU"
  CStim_HSw/1 -> Demux4/1
  Demux4/1 -> Divide12/2  "Stim_CHFL"
  Demux4/2 -> Divide22/2  "Stim_CGLU"
  Mux3/1 -> S_M4 [HFL GLU HAM]/1
  Demux1/5 -> Divide21/2  "SGainGLU_HAM"
  Divide21/1 -> Mux3/3  "HAM"
  Demux4/3 -> Divide17/2  "Stim_CHAM"
  Demux4/4 -> Divide9/2  "Stim_CRF"
  Demux1/2 -> Divide17/1  "SGainCHAM_HFL"
  Demux1/4 -> Divide9/1  "SGainCRF_GLU"
  Divide22/1 -> Sum7/1
  Sum7/1 -> Mux3/1  "HFL"
  Divide17/1 -> Sum7/2
  Divide12/1 -> Sum11/1
  Sum11/1 -> Mux3/2, Divide21/1  "GLU"
  Divide9/1 -> Sum11/2

== system nms_3Dmodel_mld/Neural Control Layer (Spinal Cord Control)/R Stance, Swing, Trans (coronal) ==
  note: DS1 (Stance -> Swing):
      | Stance Swing Transition
  note: Swing:
      | Swing Leg
  note: Full Stance:
      | PreStim, M3*F_i
  note: Stance DS1 Swing DS2
  note: FullStance Swing
  note: |------------------------------|--------------------|
  note: |--------------------|------------------------------|
  note: ContraSwing:
      | Swing Compensation
  CtrlPar : Inport
  Stance : Inport  Port=2
  CStance : Inport  Port=3
  ConI : Inport  Port=4
  ILLoad : Inport  Port=5
  CLLoad : Inport  Port=6
  S_0_St : Inport  Port=7
  S_M1 : Inport  Port=8
  S_M3 : Inport  Port=9
  S_M4 : Inport  Port=10
  S_0_Sw : Inport  Port=11
  S_M6 : Inport  Port=12
  Add : Sum  Inputs=4
  Add1 : Sum  Inputs=3
  Constant2 : Constant
  Demux{1..4} (4 alike) : Demux  Outputs=2
  Divide{1..2,4..5,12..15,24} (9 alike) : Product
  Divide31 : Product  Inputs=3
  Divide6 : Product  Inputs=3
  Logical Operator1 : Logic  Operator=NOT  AllPortsSameDT=off  OutDataTypeStr=boolean
  Logical Operator2 : Logic  Operator=NOT  AllPortsSameDT=off  OutDataTypeStr=boolean
  Logical Operator5 : Logic  Operator=NOT  AllPortsSameDT=off  OutDataTypeStr=boolean
  Logical Operator7 : Logic  AllPortsSameDT=off  OutDataTypeStr=boolean
  Mux3 : Mux  Inputs=2
  Sum1 : Sum  Inputs=|++  SaturateOnIntegerOverflow=on  InputSameDT=on  OutDataTypeStr=Inherit: Same as first input
  Sum2 : Sum  Inputs=|++  SaturateOnIntegerOverflow=on  InputSameDT=on  OutDataTypeStr=Inherit: Same as first input
  Sum4 : Sum  SaturateOnIntegerOverflow=on  InputSameDT=on  OutDataTypeStr=Inherit: Same as first input
  Sum5 : Sum  Inputs=+-|  SaturateOnIntegerOverflow=on  InputSameDT=on  OutDataTypeStr=Inherit: Same as first input
  Sum6 : Sum  Inputs=++|  SaturateOnIntegerOverflow=on  InputSameDT=on  OutDataTypeStr=Inherit: Same as first input
  S : Outport  OutputWhenDisabled=reset  InitialOutput=0
  wires:
  CStance/1 -> Logical Operator1/1
  S_M4/1 -> Divide15/2
  Logical Operator1/1 -> Divide15/1
  CLLoad/1 -> Divide1/2, Divide24/1
  Divide1/1 -> Divide31/2
  ConI/1 -> Logical Operator5/1, Divide31/1, Divide14/1  "double support"
  Stance/1 -> Logical Operator2/1, Divide6/1, Divide4/1, Logical Operator7/1
  Logical Operator2/1 -> Divide2/1, Divide5/1
  Add/1 -> Mux3/1
  Add1/1 -> Mux3/2
  S_M3/1 -> Divide6/2
  ILLoad/1 -> Divide6/3
  S_0_St/1 -> Divide4/2
  S_0_Sw/1 -> Divide5/2
  Mux3/1 -> Sum6/2
  Sum6/1 -> S/1
  S_M6/1 -> Divide31/3, Divide2/2
  Divide4/1 -> Sum4/1, [M0_St]  "M0_St (1~2)"
  Divide5/1 -> Sum4/2, [M0_Sw]  "M0_Sw (3~4)"
  Divide31/1 -> Sum1/1
  Divide2/1 -> Sum1/2
  S_M1/1 -> Divide12/2, Divide13/1  "HAB"
  Divide12/1 -> Sum2/1
  Divide13/1 -> Divide14/2
  Divide14/1 -> Sum2/2
  Logical Operator5/1 -> Logical Operator7/2
  Logical Operator7/1 -> Divide12/1  "single stance"
  Divide24/1 -> Sum5/2
  Constant2/1 -> Sum5/1
  Sum5/1 -> Divide13/2
  CtrlPar/1 -> Demux4/1  "Tr_Sw"
  Demux4/1 -> Divide24/2  "Tr_St_sup"
  Demux4/2 -> Divide1/1  "Tr_Sw"
  Sum2/1 -> [M1_HAB]
  Divide6/1 -> Demux3/1
  Demux3/1 -> [M3_HAB]
  Demux3/2 -> [M3_HAD]
  Divide15/1 -> Demux1/1
  Demux1/1 -> [M4_HAB]
  Demux1/2 -> [M4_HAD]
  Demux2/1 -> [M6_HAB]
  Demux2/2 -> [M6_HAD]
  Sum1/1 -> Demux2/1
  Sum4/1 -> Sum6/1
  [M1_HAB] -> Add/1
  [M3_HAB] -> Add/2
  [M3_HAD] -> Add1/1
  [M4_HAB] -> Add/3
  [M6_HAB] -> Add/4
  [M4_HAD] -> Add1/2
  [M6_HAD] -> Add1/3

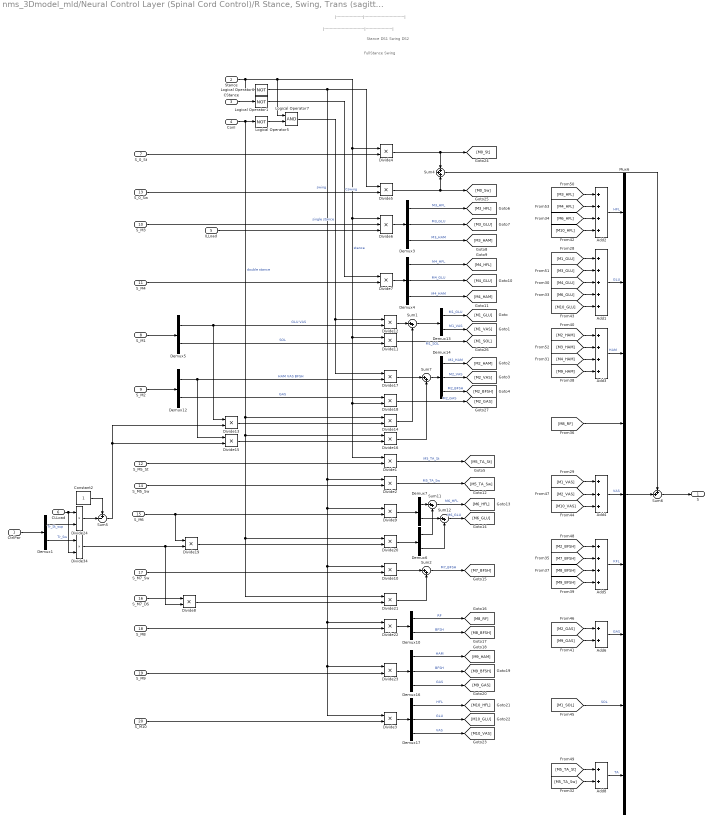
== system nms_3Dmodel_mld/Neural Control Layer (Spinal Cord Control)/R Stance, Swing, Trans (sagittal) ==
  note: Stance DS1 Swing DS2
  note: FullStance Swing
  note: |------------------------------|--------------------|
  note: |--------------------|------------------------------|
  CtrlPar : Inport
  Stance : Inport  Port=2
  CStance : Inport  Port=3
  ConI : Inport  Port=4
  ILLoad : Inport  Port=5
  CLLoad : Inport  Port=6
  S_0_St : Inport  Port=7
  S_M1 : Inport  Port=8
  S_M2 : Inport  Port=9
  S_M3 : Inport  Port=10
  S_M4 : Inport  Port=11
  S_M5_St : Inport  Port=12
  S_0_Sw : Inport  Port=13
  S_M5_Sw : Inport  Port=14
  S_M6 : Inport  Port=15
  S_M7_DS : Inport  Port=16
  S_M7_Sw : Inport  Port=17
  S_M8 : Inport  Port=18
  S_M9 : Inport  Port=19
  S_M10 : Inport  Port=20
  Add1 : Sum  Inputs=5
  Add2 : Sum  Inputs=4
  Add3 : Sum  Inputs=4
  Add4 : Sum  Inputs=3
  Add5 : Sum  Inputs=4
  Add6 : Sum  Inputs=2
  Add8 : Sum  Inputs=2
  Constant2 : Constant
  Demux{1,6..7,10,13} (5 alike) : Demux  Outputs=2
  Demux12 : Demux  Outputs=[3 1]
  Demux{3..4,14,16..17} (5 alike) : Demux  Outputs=3
  Demux5 : Demux  Outputs=[2 1]
  Divide{1..5,7..24,34} (24 alike) : Product
  Divide6 : Product  Inputs=3
  Logical Operator1 : Logic  Operator=NOT  AllPortsSameDT=off  OutDataTypeStr=boolean
  Logical Operator5 : Logic  Operator=NOT  AllPortsSameDT=off  OutDataTypeStr=boolean
  Logical Operator6 : Logic  Operator=NOT  AllPortsSameDT=off  OutDataTypeStr=boolean
  Logical Operator7 : Logic  AllPortsSameDT=off  OutDataTypeStr=boolean
  Mux6 : Mux  Inputs=9
  Sum{1..2,7,11..12} (5 alike) : Sum  Inputs=|++  SaturateOnIntegerOverflow=on  InputSameDT=on  OutDataTypeStr=Inherit: Same as first input
  Sum4 : Sum  Inputs=+++  SaturateOnIntegerOverflow=on  InputSameDT=on  OutDataTypeStr=Inherit: Same as first input
  Sum5 : Sum  Inputs=+-|  SaturateOnIntegerOverflow=on  InputSameDT=on  OutDataTypeStr=Inherit: Same as first input
  Sum6 : Sum  Inputs=++|  SaturateOnIntegerOverflow=on  InputSameDT=on  OutDataTypeStr=Inherit: Same as first input
  S : Outport  OutputWhenDisabled=reset  InitialOutput=0
  wires:
  CtrlPar/1 -> Demux1/1
  Stance/1 -> Logical Operator6/1, Logical Operator7/1, Divide4/1, Divide11/1, Divide18/2, Divide1/1, Divide6/1  "stance"
  ConI/1 -> Logical Operator5/1, Divide14/1, Divide16/1, Divide20/1, Divide21/1  "double stance"
  Logical Operator5/1 -> Logical Operator7/2
  S_M4/1 -> Divide7/2
  CStance/1 -> Logical Operator1/1
  Logical Operator1/1 -> Divide7/1  "Cswing"
  Demux1/1 -> Divide24/2  "Tr_St_sup"
  Divide24/1 -> Sum5/2
  Constant2/1 -> Sum5/1
  CLLoad/1 -> Divide24/1, Divide34/2
  Demux4/1 -> [M4_HFL]  "M4_HFL"
  Add2/1 -> Mux6/1  "HFL"
  Add1/1 -> Mux6/2  "GLU"
  Demux4/2 -> [M4_GLU]  "M4_GLU"
  Add3/1 -> Mux6/3  "HAM"
  Demux4/3 -> [M4_HAM]  "M4_HAM"
  Add4/1 -> Mux6/5  "VAS"
  Add5/1 -> Mux6/6  "KFL"
  Add6/1 -> Mux6/7  "GAS"
  Add8/1 -> Mux6/9  "TA"
  Demux1/2 -> Divide34/1  "Tr_Sw"
  Divide7/1 -> Demux4/1
  Logical Operator7/1 -> Divide12/1, Divide17/1  "single stance"
  Divide34/1 -> Divide19/2, Divide8/2
  Logical Operator6/1 -> Divide5/1, Divide2/1, Divide9/1, Divide10/1, Divide3/1, Divide23/1, Divide22/1  "swing"
  Mux6/1 -> Sum6/2
  Sum6/1 -> S/1
  Sum4/1 -> Sum6/1
  S_0_Sw/1 -> Divide5/2
  S_0_St/1 -> Divide4/2
  Divide5/1 -> Sum4/3, [M0_Sw]
  Divide4/1 -> Sum4/1, [M0_St]
  S_M1/1 -> Demux5/1
  S_M2/1 -> Demux12/1
  Demux5/1 -> Divide12/2, Divide13/1  "GLU VAS"
  Demux5/2 -> Divide11/2  "SOL"
  Divide12/1 -> Sum1/1
  Divide13/1 -> Divide14/2
  Divide14/1 -> Sum1/2
  Divide16/1 -> Sum7/2
  Divide15/1 -> Divide16/2
  Sum1/1 -> Demux13/1
  Demux13/1 -> [M1_GLU]  "M1_GLU"
  Demux13/2 -> [M1_VAS]  "M1_VAS"
  Demux12/1 -> Divide17/2, Divide15/1  "HAM VAS BFSH"
  Divide17/1 -> Sum7/1
  Sum7/1 -> Demux14/1
  Demux14/1 -> [M2_HAM]  "M2_HAM"
  Demux14/2 -> [M2_VAS]  "M2_VAS"
  Demux14/3 -> [M2_BFSH]  "M2_BFSH"
  Demux12/2 -> Divide18/1  "GAS"
  Divide18/1 -> [M2_GAS]  "M2_GAS"
  S_M5_St/1 -> Divide1/2
  Divide1/1 -> [M5_TA_St]  "M5_TA_St"
  Divide11/1 -> [M1_SOL]  "M1_SOL"
  S_M3/1 -> Divide6/2
  ILLoad/1 -> Divide6/3
  Divide6/1 -> Demux3/1
  Demux3/1 -> [M3_HFL]  "M3_HFL"
  Demux3/2 -> [M3_GLU]  "M3_GLU"
  Demux3/3 -> [M3_HAM]  "M3_HAM"
  S_M5_Sw/1 -> Divide2/2
  Divide2/1 -> [M5_TA_Sw]  "M5_TA_Sw"
  S_M6/1 -> Divide9/2, Divide19/1
  Divide9/1 -> Demux7/1
  Demux7/2 -> Sum12/1
  Divide20/1 -> Demux6/1
  Demux6/1 -> Sum11/2
  Demux6/2 -> Sum12/2
  Demux7/1 -> Sum11/1
  Divide19/1 -> Divide20/2
  Sum11/1 -> [M6_HFL]  "M6_HFL"
  Sum12/1 -> [M6_GLU]  "M6_GLU"
  Divide10/1 -> Sum2/1
  Divide21/1 -> Sum2/2
  Sum5/1 -> Divide13/2, Divide15/2
  S_M7_Sw/1 -> Divide10/2
  Divide8/1 -> Divide21/2
  S_M7_DS/1 -> Divide8/1
  Sum2/1 -> [M7_BFSH]  "M7_BFSH"
  S_M8/1 -> Divide22/2
  Divide22/1 -> Demux10/1
  S_M9/1 -> Divide23/2
  Divide23/1 -> Demux16/1
  S_M10/1 -> Divide3/2
  Divide3/1 -> Demux17/1
  Demux10/2 -> [M8_BFSH]  "BFSH"
  Demux10/1 -> [M8_RF]  "RF"
  Demux16/1 -> [M9_HAM]  "HAM"
  Demux16/2 -> [M9_BFSH]  "BFSH"
  Demux16/3 -> [M9_GAS]  "GAS"
  Demux17/1 -> [M10_HFL]  "HFL"
  Demux17/2 -> [M10_GLU]  "GLU"
  Demux17/3 -> [M10_VAS]  "VAS"
  [M1_GLU] -> Add1/1
  [M3_GLU] -> Add1/2
  [M4_GLU] -> Add1/3
  [M6_GLU] -> Add1/4
  [M10_GLU] -> Add1/5
  [M1_VAS] -> Add4/1
  [M2_HAM] -> Add3/1
  [M2_VAS] -> Add4/2
  [M2_BFSH] -> Add5/1
  [M2_GAS] -> Add6/1
  [M3_HFL] -> Add2/1
  [M3_HAM] -> Add3/2
  [M4_HFL] -> Add2/2
  [M4_HAM] -> Add3/3
  [M5_TA_St] -> Add8/1
  [M5_TA_Sw] -> Add8/2
  [M6_HFL] -> Add2/3
  [M7_BFSH] -> Add5/2
  [M9_BFSH] -> Add5/4
  [M8_BFSH] -> Add5/3
  [M8_RF] -> Mux6/4
  [M9_HAM] -> Add3/4
  [M9_GAS] -> Add6/2
  [M10_HFL] -> Add2/4
  [M10_VAS] -> Add4/3
  [M1_SOL] -> Mux6/8  "SOL"

== system nms_3Dmodel_mld/Neural Control Layer (Spinal Cord Control)/R Swing Phase (coronal) ==
  note: Left Swing Phase Control
  note: M6: swing hip
  CtrlPar : Inport
  R_a_tgt : Inport  Port=2
  LceHAD : Inport  Port=3
  LceHAB : Inport  Port=4
  Enable : EnablePort  StatesWhenEnabling=reset  ZeroCross=off
  Constant1 : Constant
  Constant5 : Constant
  Demux4 : Demux  Outputs=6
  Divide{1..2,5,22} (4 alike) : Product
  Mux1 : Mux  Inputs=2
  R_parSwPreS : Selector  InputPortWidth=R_Sw_i  IndexOptions=Index vector (dialog)  Indices=R_parSw_PreS_i  OutputSizes=1
  R_parSw_M6 : Selector  InputPortWidth=R_Sw_i  IndexOptions=Index vector (dialog)  Indices=R_parSw_M6_i  OutputSizes=1
  Sum1 : Sum  Inputs=-+|  SaturateOnIntegerOverflow=on  InputSameDT=on  OutDataTypeStr=Inherit: Same as first input
  Sum10 : Sum  Inputs=++|  SaturateOnIntegerOverflow=on  InputSameDT=on  OutDataTypeStr=Inherit: Same as first input
  Sum13 : Sum  Inputs=|+-  SaturateOnIntegerOverflow=on  InputSameDT=on  OutDataTypeStr=Inherit: Same as first input
  Sum2 : Sum  Inputs=-+|  SaturateOnIntegerOverflow=on  InputSameDT=on  OutDataTypeStr=Inherit: Same as first input
  Sum3 : Sum  Inputs=+-|  SaturateOnIntegerOverflow=on  InputSameDT=on  OutDataTypeStr=Inherit: Same as first input
  Sum4 : Sum  Inputs=|+-  SaturateOnIntegerOverflow=on  InputSameDT=on  OutDataTypeStr=Inherit: Same as first input
  positive half1 : Saturate  UpperLimit=inf  LowerLimit=0  ZeroCross=off
  positive half2 : Saturate  UpperLimit=inf  LowerLimit=0  ZeroCross=off
  S_0_Sw : Outport  OutputWhenDisabled=reset  InitialOutput=0
  S_M6 : Outport  Port=2  OutputWhenDisabled=reset  InitialOutput=0
  wires:
  R_parSwPreS/1 -> S_0_Sw/1
  CtrlPar/1 -> R_parSwPreS/1, R_parSw_M6/1
  R_parSw_M6/1 -> Demux4/1
  Constant5/1 -> Sum10/1
  Demux4/2 -> Sum13/2  "aRef_HAB"
  Sum13/1 -> Divide22/2
  Demux4/1 -> Divide22/1  "a2lopt_HAB"
  Divide22/1 -> Sum10/2
  Sum10/1 -> Sum1/1  "lceOffHAB"
  Sum1/1 -> positive half2/1
  positive half2/1 -> Divide5/1
  Demux4/3 -> Divide5/2  "LGain_HAB"
  Constant1/1 -> Sum3/1
  R_a_tgt/1 -> Sum4/1, Sum13/1
  Demux4/5 -> Sum4/2  "aRef_HAD"
  Sum4/1 -> Divide1/2
  Demux4/4 -> Divide1/1  "a2lopt_HAD"
  Divide1/1 -> Sum3/2
  Sum3/1 -> Sum2/1  "lceOffHAD"
  Sum2/1 -> positive half1/1
  positive half1/1 -> Divide2/1
  Demux4/6 -> Divide2/2  "LGain_HAD"
  LceHAB/1 -> Sum1/2
  LceHAD/1 -> Sum2/2
  Divide5/1 -> Mux1/1  "HAB"
  Divide2/1 -> Mux1/2  "HAD"
  Mux1/1 -> S_M6/1
